simulink model "sim_pil_target_BLDC_Commutation_s32k1xx"  (Simulink 9.0)
settings: Solver=FixedStepDiscrete  StartTime=0.0  StopTime=1.2  FixedStep=0.1  RelTol=1e-3  EnableMultiTasking=on
InitFcn:
  | mbd_s32k_consistency_checks(bdroot(gcs));
undefined symbols (not defined in the file): LQFP
libraries: mbd_s32k1xx_ec_toolbox x2
settings Model: Creator=NXP MBDT Team  LastModifiedBy=nxf35172
settings DataIOCC: ExternalInput=off  InitialState=off  LimitDataPoints=on  SaveOutput=off  SignalLogging=off  SaveTime=off
settings OptimizationCC: DefaultParameterBehavior=Inlined  LifeSpan=1
settings DebuggingCC: UnderspecifiedInitializationDetection=Simplified  MergeDetectMultiDrivingBlocksExec=error  SolverPrmCheckMsg=warning  InheritedTsInSrcMsg=none  SingleTaskRateTransMsg=error  UnconnectedInputMsg=error  UnconnectedOutputMsg=error  UnconnectedLineMsg=error  AllowSymbolicDim=off  UnknownTsInhSupMsg=error
settings HardwareCC: ProdLargestAtomicInteger=Long  ProdLargestAtomicFloat=Double  ProdIntDivRoundTo=Zero  ProdEndianess=LittleEndian  ProdHWDeviceType=ARM Compatible->ARM Cortex
settings SFSimCC: MATLABDynamicMemAlloc=off
settings RTWCC: SystemTargetFile=mbd_s32k.tlc  MakeCommand=mbd_s32k_make_rtw COPY_MDLREF_INCLUDES=0  TemplateMakefile=mbd_s32k.tmf  Description=Model Based Design Toolbox S32K14x Code Generation Target
settings CodeAppCC: IgnoreCustomStorageClasses=off  MaxIdLength=63
settings STFCustomTargetCC: CombineOutputUpdateFcns=on  SuppressErrorStatus=on  ERTCustomFileBanners=on  SupportAbsoluteTime=off  SupportContinuousTime=off  SupportNonInlinedSFcns=off  RemoveResetFunc=on  MATLABClassNameForMDSCustomization=Simulink.SoftwareTarget.ERTCustomization  GRTInterface=off  SystemTargetFile=mbd_s32k14.tlc
settings ERTTargetCC: MultiwordLength=2048  ParMdlRefBuildCompliant=off  CompOptLevelCompliant=off  ConcurrentExecutionCompliant=off  SuppressErrorStatus=on  SupportAbsoluteTime=off  ModelStepFunctionPrototypeControlCompliant=off  CPPClassGenCompliant=off  UseToolchainInfoCompliant=off  InlinedParameterPlacement=NonHierarchical  ERTCustomFileTemplate=example_file_process.tlc  ConvertIfToSwitch=off  SuppressUnreachableDefaultCases=off

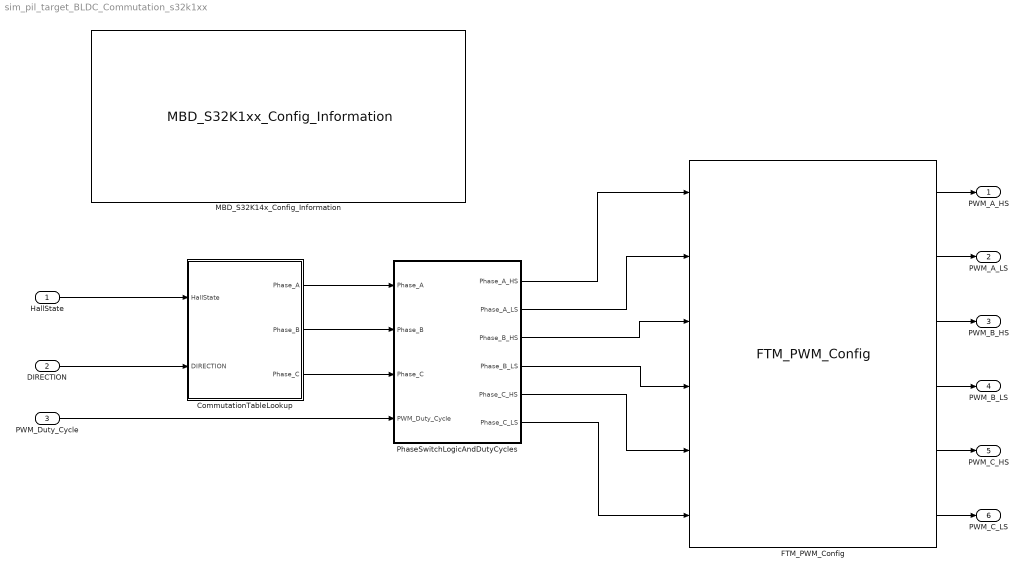
== system sim_pil_target_BLDC_Commutation_s32k1xx ==
  HallState : Inport
  DIRECTION : Inport  Port=2
  PWM_Duty_Cycle : Inport  Port=3
  CommutationTableLookup : Stateflow chart  TreatAsAtomicUnit=on
  FTM_PWM_Config : mbd_s32k1xx_ec_toolbox/Motor Control Blocks/FTM Blocks/FTM_PWM_Config  Priority=1  ftmModule=0  ftmMode=Center-Aligned PWM  ftmSourceClock=80 MHz  swcontrol_enable=off  chan0En=on  chan0Type=Independent  chan2En=on  chan2Type=Independent  chan4En=on  chan4Type=Independent  chan6En=off  chan6Type=Independent  ftmPwmUnits=Hz  outFrequency=1000  ftmPeriod=20000  ftmPrescaler=Divide by 4  deadtimeUnits=Nanoseconds  deadtimeNs=0  deadtimeTicks=0  deadtimePrescaler=Divide by 1  dutyCycleCh0=0.26  dutyCycleCh1=0.25  dutyCycleCh2=0.25  dutyCycleCh3=0.25  dutyCycleCh4=0.25  dutyCycleCh5=0.25  dutyCycleCh6=0.25  dutyCycleCh7=0.25  dutyCycleSim=on  startAfterInit=on  showAdvOpt=on  pinFtmCh0=PTB12: [FTM0_CH0 | FTM Channel]  pinFtmCh1=None  pinPolCh0=Active Low  pinPolCh1=Active Low  outputComplem0=Main duplicated  outputLevel0=Low  outputLevel1=Low  pinFtmCh2=PTC2: [FTM0_CH2 | FTM Channel]  pinFtmCh3=None  pinPolCh2=Active Low  pinPolCh3=Active Low  outputComplem2=Main duplicated  outputLevel2=Low  outputLevel3=Low  pinFtmCh4=PTB4: [FTM0_CH4 | FTM Channel]  pinFtmCh5=None  pinPolCh4=Active Low  pinPolCh5=Active Low  outputComplem4=Main duplicated  outputLevel4=Low  outputLevel5=Low  pinFtmCh6=PTA17: [FTM0_CH6 | FTM Channel]  pinFtmCh7=None  pinPolCh6=Active Low  pinPolCh7=Active Low  outputComplem6=Main duplicated  outputLevel6=Low  outputLevel7=Low  initTrigger=off  chTrigger0=off  chTrigger1=off  chTrigger2=off  chTrigger3=off  chTrigger4=off  chTrigger5=off  chTrigger6=off  chTrigger7=off  mcuTargetUpdate=on  pwmSyncTrg=Software trigger  pwmSyncHwRouting=TRGMUX_FTM7  pwmSyncTrg0=off  pwmSyncTrg1=off  pwmSyncTrg2=off  pwmSyncAutoClear=on  pwmSyncMinLoad=on  pwmSyncMaxLoad=on  pwmSyncInvert=System Clock  pwmSyncOutControl=System Clock  pwmSyncOutMask=System Clock  pwmSyncCounterInitial=System Clock  pwmSyncPoints=Update now  reloadEnable=off  reloadPriority=15  reloadHalfCycle=off  reloadHCR=0  reloadFrequency=0  chnMatch0=off  chnMatch1=off  chnMatch2=off  chnMatch3=off  chnMatch4=off  chnMatch5=off  chnMatch6=off  chnMatch7=off  pwmFaultProtection=off  pwmFaultInterrupt=off  pwmFaultClearing=Fault control disabled  pwmFaultPinState=Safe Value  pwmFaultFilterValue=0  pwmFaultPriority=15  fault_disen_0=off  fault_filter_0=off  fault_polarity_0=Active High  fault_disen_1=off  fault_filter_1=off  fault_polarity_1=Active high  fault_disen_2=off  fault_filter_2=off  fault_polarity_2=Active high  fault_disen_3=off  fault_filter_3=off  fault_polarity_3=Active high  fault_pin_0=None  fault_pin_1=None  fault_pin_2=None  fault_pin_3=None
  MBD_S32K14x_Config_Information : mbd_s32k1xx_ec_toolbox/MBD_S32K1xx_Config_Information  mbdt_ver=0  disp_str=|  config_params=[]  mcu_target_name=S32K144  mcu_target_package=100-LQFP  mcu_target_sram_size=64KB  mcu_system_clock_freq=80  mcu_xtal_freq=External 8  mcu_steptick_timer=LPIT Channel 0  mcu_steptick_prio=15  ds_import_enable=off  target_compiler=GCC  target_memory=FLASH  gcc_target_compile_opts=-mcpu=cortex-m4 -mthumb -mfloat-abi=hard -mfpu=fpv4-sp-d16 -O1 -g -gstrict-dwarf  gcc_target_assemble_opts=-mcpu=cortex-m4 -mthumb -mfloat-abi=hard -mfpu=fpv4-sp-d16 -g  gcc_target_link_opts=-mcpu=cortex-m4 -mthumb -mfloat-abi=hard -mfpu=fpv4-sp-d16  gcc_target_default_lcf=on  gcc_target_user_lcf=S32K144_64_flash.ld  ghs_target_compile_opts=-cpu=cortexm4f -thumb -DARM_MATH_CM4 -fpu=vfpv4_d16 -fsingle -Ogeneral -Wundef -Wimplicit-int -Wshadow -Wtrigraphs --no_commons --gnu_asm -gnu99 -gdwarf-2 -G  ghs_target_assemble_opts=-cpu=cortexm4f -fpu=vfpv4_d16  ghs_target_link_opts=-cpu=cortexm4f -thumb -fpu=vfpv4_d16  ghs_target_default_lcf=on  ghs_target_user_lcf=S32K144_64_flash.ld  iar_target_compile_opts=--cpu=Cortex-M4F --thumb --fpu=VFPv4_sp -Ol -e --debug --dlib_config normal  iar_target_assemble_opts=--cpu Cortex-M4F --thumb --fpu VFPv4_sp  iar_target_link_opts=--no_exceptions --vfe --inline  iar_target_default_lcf=on  iar_target_user_lcf=S32K144_64_flash.icf  pil_download_enable=on  rbl_download_enable=off  rbl_start_delay=5000000  rbl_download_interface=OpenSDA  rbl_restart_request=off  rbl_com_port=Custom  rbl_com_port_custom=COM1  pil_download_rate=57600  pil_opensda_drive=Custom  pil_opensda_drive_custom=D  pil_uart_instance=1  pil_uart_rx=PTC6: [LPUART1_RX | Receive]  pil_uart_tx=PTC7: [LPUART1_TX | Transmit]  FTM_PWM_PcrCheckEnDis=on  FTM_Input_Edge_Inputs_PcrCheckEnDis=on  FTM_Dual_Edge_Inputs_PcrCheckEnDis=on  FTM_Quadrature_Inputs_PcrCheckEnDis=on  FTM_Hall_Sensor_Inputs_PcrCheckEnDis=on  LPTMR_PcrCheckEnDis=on  PIT_PcrCheckEnDis=on  RTC_PcrCheckEnDis=on  FlexCAN_PcrCheckEnDis=on  LIN_PcrCheckEnDis=on  FlexIO_PcrCheckEnDis=on  LPI2C_PcrCheckEnDis=on  LPSPI_PcrCheckEnDis=on  LPUART_PcrCheckEnDis=on  CMP_PcrCheckEnDis=on  GPIO_OutputPcrCheckEnDis=on  GPIO_InputPcrCheckEnDis=on  SBC_PcrCheckEnDis=on  AMMCLIB_PcrCheckEnDis=on  FM_PcrCheckEnDis=on  Profile_PcrCheckEnDis=on  ConfigParams_PcrCheckEnDis=on  ModelRef_PcrCheckEnDis=on  PDB0_PcrCheckEnDis=on  CSEc_PcrCheckEnDis=on  eDMA_PcrCheckEnDis=on  ADC_PcrCheckEnDis=on  WDOG_PcrCheckEnDis=on
      | Target : S32K144-64KB_SRAM
      | Package : 100-pin
      | System clock : 80 MHz
      | XTAL clock : External 8 MHz
      | Compiler : GCC
      | Target Type : FLASH
      | Processor-In-Loop : (COM1, 115200, OpenSDA: E)
      | Step Tick Interrupt Priority : 15
  PhaseSwitchLogicAndDutyCycles : Stateflow chart  TreatAsAtomicUnit=on
  PWM_A_HS : Outport
  PWM_A_LS : Outport  Port=2
  PWM_B_HS : Outport  Port=3
  PWM_B_LS : Outport  Port=4
  PWM_C_HS : Outport  Port=5
  PWM_C_LS : Outport  Port=6
  wires:
  HallState/1 -> CommutationTableLookup/1(HallState)
  CommutationTableLookup/2(Phase_B) -> PhaseSwitchLogicAndDutyCycles/2(Phase_B)
  CommutationTableLookup/1(Phase_A) -> PhaseSwitchLogicAndDutyCycles/1(Phase_A)
  DIRECTION/1 -> CommutationTableLookup/2(DIRECTION)
  PWM_Duty_Cycle/1 -> PhaseSwitchLogicAndDutyCycles/4(PWM_Duty_Cycle)
  CommutationTableLookup/3(Phase_C) -> PhaseSwitchLogicAndDutyCycles/3(Phase_C)
  PhaseSwitchLogicAndDutyCycles/1(Phase_A_HS) -> FTM_PWM_Config/1
  PhaseSwitchLogicAndDutyCycles/2(Phase_A_LS) -> FTM_PWM_Config/2
  PhaseSwitchLogicAndDutyCycles/3(Phase_B_HS) -> FTM_PWM_Config/3
  PhaseSwitchLogicAndDutyCycles/4(Phase_B_LS) -> FTM_PWM_Config/4
  PhaseSwitchLogicAndDutyCycles/5(Phase_C_HS) -> FTM_PWM_Config/5
  PhaseSwitchLogicAndDutyCycles/6(Phase_C_LS) -> FTM_PWM_Config/6
  FTM_PWM_Config/6 -> PWM_C_LS/1
  FTM_PWM_Config/5 -> PWM_C_HS/1
  FTM_PWM_Config/4 -> PWM_B_LS/1
  FTM_PWM_Config/3 -> PWM_B_HS/1
  FTM_PWM_Config/2 -> PWM_A_LS/1
  FTM_PWM_Config/1 -> PWM_A_HS/1

== stateflow chart CommutationTableLookup ==
  (junction 11) -> (junction 10) [order 1] : /*If Direction is Negative */
      | [DIRECTION < 0]
  (default) -> (junction 11)
  (junction 10) -> (junction 12) : {
      |    Phase_A = ccwTable[HallState][0];
      |    Phase_B = ccwTable[HallState][1];
      |    Phase_C = ccwTable[HallState][2];
      | }
  (junction 11) -> (junction 13) [order 2] : {
      |    Phase_A = cwTable[HallState][0];
      |    Phase_B = cwTable[HallState][1];
      |    Phase_C = cwTable[HallState][2];
      | }
  (junction 13) -> (junction 12)
  data: cwTable constant uint8 size=[8 3] =[0 0 0; 2 1 0; 0 2 1; 2 0 1; 1 0 2; 0 1 2; 1 2 0; 0 0 0]; HallState input uint8; Phase_A output uint8; Phase_B output uint8; Phase_C output uint8; ccwTable constant uint8 size=[8 3] =[0 0 0; 1 2 0; 0 1 2; 1 0 2; 2 0 1; 0 2 1; 2 1 0; 0 0 0]; DIRECTION input single

== stateflow chart PhaseSwitchLogicAndDutyCycles ==
  settings: sampleTime=0.500
  note: Phase States:
      | 0 = NC
      | 1 = -Vdcb
      | 2 = +Vdcb
  (default) -> (junction 32)
  (junction 32) -> (junction 33) [order 1] : /*check for phase state 0 */
      | [Phase_A == 0]
      | /*set output for state 0 */
      | {Phase_A_HS = 0; Phase_A_LS =0;}
  (junction 32) -> (junction 34) [order 2]
  (junction 33) -> (junction 35)
  (junction 34) -> (junction 35) [order 1] : /*check for phase state 1 */
      | [Phase_A == 1]
      | /*set output for state 1 */
      | {Phase_A_HS = 0; Phase_A_LS = PWM_Duty_Cycle;}
  (junction 34) -> (junction 36) [order 2]
  (junction 35) -> (junction 37)
  (junction 36) -> (junction 37) [order 1] : /*check for phase state 2 */
      | [Phase_A == 2]
      | /*set output for state 2 */
      | {Phase_A_HS = 1; Phase_A_LS = 0;}
  (junction 36) -> (junction 38) [order 2]
  (junction 37) -> (junction 39)
  (junction 38) -> (junction 39)
  (junction 39) -> (junction 40) [order 1] : /*check for phase state 0 */
      | [Phase_B == 0]
      | /*set output for state 0 */
      | {Phase_B_HS = 0; Phase_B_LS = 0;}
  (junction 39) -> (junction 41) [order 2]
  (junction 40) -> (junction 42)
  (junction 41) -> (junction 42) [order 1] : /*check for phase state 1 */
      | [Phase_B == 1]
      | /*set output for state 1 */
      | {Phase_B_HS = 0; Phase_B_LS = PWM_Duty_Cycle;}
  (junction 41) -> (junction 43) [order 2]
  (junction 42) -> (junction 44)
  (junction 43) -> (junction 44) [order 1] : /*check for phase state 2 */
      | [Phase_B == 2]
      | /*set output for state 2 */
      | {Phase_B_HS = 1; Phase_B_LS = 0;}
  (junction 43) -> (junction 45) [order 2]
  (junction 44) -> (junction 46)
  (junction 45) -> (junction 46)
  (junction 46) -> (junction 47) [order 1] : /*check for phase state 0 */
      | [Phase_C == 0]
      | /*set output for state 0 */
      | {Phase_C_HS = 0; Phase_C_LS = 0;}
  (junction 46) -> (junction 48) [order 2]
  (junction 47) -> (junction 49)
  (junction 48) -> (junction 49) [order 1] : /*check for phase state 1 */
      | [Phase_C == 1]
      | /*set output for state 1 */
      | {Phase_C_HS = 0; Phase_C_LS = PWM_Duty_Cycle;}
  (junction 48) -> (junction 50) [order 2]
  (junction 49) -> (junction 51)
  (junction 50) -> (junction 51) [order 1] : /*check for phase state 2 */
      | [Phase_C == 2]
      | /*set output for state 2 */
      | {Phase_C_HS = 1; Phase_C_LS = 0;}
  (junction 50) -> (junction 52) [order 2]
  (junction 51) -> (junction 53)
  (junction 52) -> (junction 53)
  data: Phase_A input uint8; Phase_B input uint8; Phase_C input uint8; Phase_A_HS output single; Phase_A_LS output single; Phase_B_HS output single; Phase_B_LS output single; Phase_C_HS output single; Phase_C_LS output single; PWM_Duty_Cycle input single [0..100]
